simulink subsystem "RoboticArmGeneral7DOF"  (R2022a)
settings: Solver=VariableStepAuto  StartTime=0.0  StopTime=10.0  RelTol=1e-3
undefined symbols (not defined in the file): armAttachOffset, smiData, X, Y, Z
libraries: nesl_utility x227, sm_lib x75
(part 1 of 3)
settings Model: Creator=Andy  LastModifiedBy=Andy

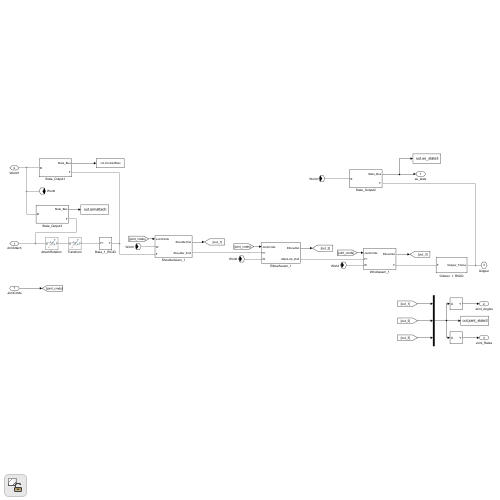
[thumbnail: Simulink's stored preview of the top-level diagram]
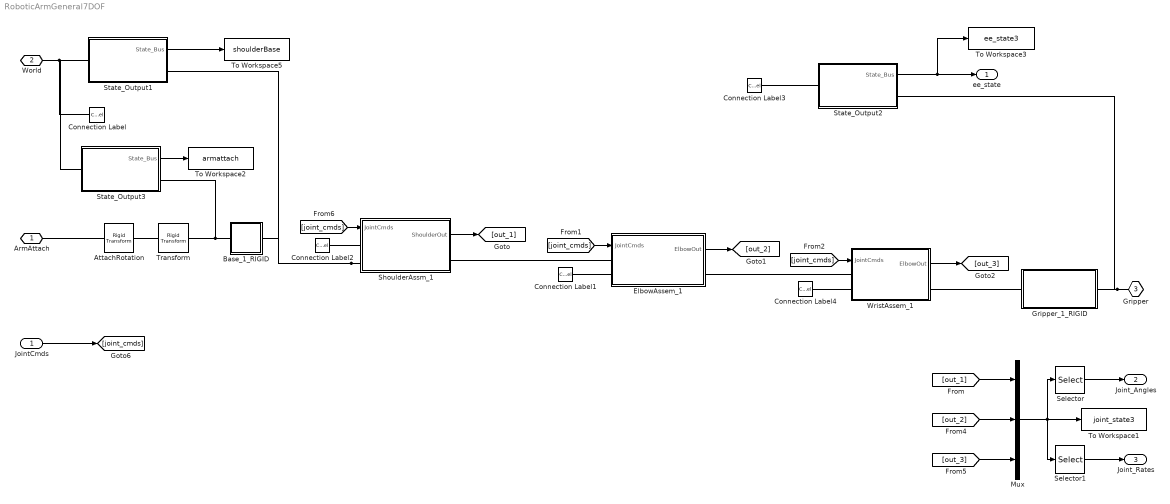
== system RoboticArmGeneral7DOF ==
  JointCmds : Inport
  AttachRotation : sm_lib/Frames and Transforms/Rigid Transform  TranslationMethod=Cartesian  TranslationStandardOffset=0  TranslationLengthUnit=m  TranslationStandardAxis=+Z  TranslationCartesianOffset=armAttachOffset(1).translation  TranslationROffset=0  TranslationROffsetUnits=m  TranslationZOffset=0  TranslationZOffsetUnits=m  TranslationThetaOffset=0  TranslationThetaOffsetUnits=deg  RotationMethod=RotationSequence  RotationAngleUnits=rad  RotationStandardAxis=+Z  RotationAngle=smiData.RigidTransform(21).angle  RotationArbitraryAxis=smiData.RigidTransform(21).axis  FollAlignAxisA=+X  BaseAlignAxisA=+Y  FollAlignAxisB=+Y  BaseAlignAxisB=+Z  RotationSequenceAxes=BaseAxes  RotationSequence=ZYX  RotationSequenceAngles=armAttachOffset(1).orientation  RotationSequenceAnglesUnits=rad  RotationMatrix=[1 0 0; 0 1 0; 0 0 1]
  Base_1_RIGID : Subsystem
  Connection Label{,1..4} (5 alike) : ConnectionLabel  Label=World
  ElbowAssem_1 : Subsystem
  Gripper_1_RIGID : Subsystem
  Mux : Mux  Inputs=3
  Selector : Selector  InputPortWidth=28  IndexOptions=Index vector (dialog)  Indices=[1 5 9 13 17 21 25]  OutputSizes=1
  Selector1 : Selector  InputPortWidth=28  IndexOptions=Index vector (dialog)  Indices=[2 6 10 14 18 22 26]  OutputSizes=1
  ShoulderAssm_1 : Subsystem
  State_Output1 : Subsystem
  State_Output2 : Subsystem
  State_Output3 : Subsystem
  To Workspace1 : ToWorkspace  VariableName=joint_state3  SaveFormat=Timeseries  SampleTime=-1
  To Workspace2 : ToWorkspace  VariableName=armattach  SaveFormat=Timeseries  SampleTime=-1
  To Workspace3 : ToWorkspace  VariableName=ee_state3  SaveFormat=Timeseries  SampleTime=-1
  To Workspace5 : ToWorkspace  VariableName=shoulderBase  SaveFormat=Timeseries  SampleTime=-1
  Transform : sm_lib/Frames and Transforms/Rigid Transform  TranslationMethod=Cartesian  TranslationStandardOffset=0  TranslationLengthUnit=m  TranslationStandardAxis=+Z  TranslationCartesianOffset=smiData.RigidTransform(26).translation  TranslationROffset=0  TranslationROffsetUnits=m  TranslationZOffset=0  TranslationZOffsetUnits=m  TranslationThetaOffset=0  TranslationThetaOffsetUnits=deg  RotationMethod=ArbitraryAxis  RotationAngleUnits=rad  RotationStandardAxis=+Z  RotationAngle=smiData.RigidTransform(26).angle  RotationArbitraryAxis=smiData.RigidTransform(26).axis  FollAlignAxisA=+X  BaseAlignAxisA=+Y  FollAlignAxisB=+Y  BaseAlignAxisB=+Z  RotationSequenceAxes=FollowerAxes  RotationSequence=XYX  RotationSequenceAngles=[0 0 0]  RotationSequenceAnglesUnits=deg  RotationMatrix=[1 0 0; 0 1 0; 0 0 1]
  WristAssem_1 : Subsystem
  ArmAttach : PMIOPort  Side=Left
  World : PMIOPort  Port=2  Side=Left
  Gripper : PMIOPort  Port=3  Side=Right
  ee_state : Outport
  Joint_Angles : Outport  Port=2
  Joint_Rates : Outport  Port=3
  wires:
  Mux/1 -> Selector1/1, Selector/1, To Workspace1/1
  [out_2] -> Mux/2
  [out_3] -> Mux/3
  State_Output1/1(State_Bus) -> To Workspace5/1
  Selector1/1 -> Joint_Rates/1
  ShoulderAssm_1/1(ShoulderOut) -> [out_1]
  [joint_cmds] -> ElbowAssem_1/1(JointCmds)
  Selector/1 -> Joint_Angles/1
  State_Output2/1(State_Bus) -> ee_state/1, To Workspace3/1
  [out_1] -> Mux/1
  [joint_cmds] -> WristAssem_1/1(JointCmds)
  JointCmds/1 -> [joint_cmds]
  ElbowAssem_1/1(ElbowOut) -> [out_2]
  State_Output3/1(State_Bus) -> To Workspace2/1
  [joint_cmds] -> ShoulderAssm_1/1(JointCmds)
  WristAssem_1/1(ElbowOut) -> [out_3]
  connections:
  ShoulderAssm_1/LConn2 -- State_Output1/RConn1 -- Base_1_RIGID/RConn1
  World/RConn1 -- Connection Label/LConn1 -- State_Output3/LConn1 -- State_Output1/LConn1
  Gripper/RConn1 -- State_Output2/RConn1 -- Gripper_1_RIGID/RConn1
  State_Output3/RConn1 -- Base_1_RIGID/LConn1 -- Transform/RConn1
  ArmAttach/RConn1 -- AttachRotation/LConn1
  AttachRotation/RConn1 -- Transform/LConn1
  Connection Label2/LConn1 -- ShoulderAssm_1/LConn1
  Connection Label3/LConn1 -- State_Output2/LConn1
  Connection Label4/LConn1 -- WristAssem_1/LConn2
  ElbowAssem_1/LConn1 -- ShoulderAssm_1/RConn1
  Connection Label1/LConn1 -- ElbowAssem_1/LConn2
  ElbowAssem_1/RConn1 -- WristAssem_1/LConn1
  WristAssem_1/RConn1 -- Gripper_1_RIGID/LConn1

== system RoboticArmGeneral7DOF/Base_1_RIGID ==
  ReferenceFrame : sm_lib/Frames and Transforms/Reference Frame
  Solid : sm_lib/Body Elements/File Solid  ExtGeomFileName=Base_Default_sldprt.STEP  UnitType=FromFile  ExtGeomFileUnits=m  StepReaderType=HEX  ExportConvexHullGeometry=off  InertiaType=Custom  Mass=smiData.Solid(11).mass  MassUnits=kg  CenterOfMass=smiData.Solid(11).CoM  CenterOfMassUnits=m  MomentsOfInertia=smiData.Solid(11).MoI  MomentsOfInertiaUnits=kg*m^2  ProductsOfInertia=smiData.Solid(11).PoI  ProductsOfInertiaUnits=kg*m^2  BasedOnType=DensityFromFile  Density=1000  DensityUnits=kg/m^3  DoExposeReferenceFrame=on  SerializedFrames=<Frames/>  GraphicType=FromGeometry  MarkerShape=Sphere  MarkerSize=10  GraphicVisPropType=SimpleVisualProperties  GraphicDiffuseColor=smiData.Solid(11).color  GraphicSpecularColor=[0.5 0.5 0.5 1.0]  GraphicAmbientColor=[0.15 0.15 0.15 1.0]  GraphicEmissiveColor=[0.0 0.0 0.0 1.0]  GraphicShininess=75  GraphicOpacity=smiData.Solid(11).opacity
  Transform : sm_lib/Frames and Transforms/Rigid Transform  TranslationMethod=Cartesian  TranslationStandardOffset=0  TranslationLengthUnit=m  TranslationStandardAxis=+Z  TranslationCartesianOffset=smiData.RigidTransform(16).translation  TranslationROffset=0  TranslationROffsetUnits=m  TranslationZOffset=0  TranslationZOffsetUnits=m  TranslationThetaOffset=0  TranslationThetaOffsetUnits=deg  RotationMethod=ArbitraryAxis  RotationAngleUnits=rad  RotationStandardAxis=+Z  RotationAngle=smiData.RigidTransform(16).angle  RotationArbitraryAxis=smiData.RigidTransform(16).axis  FollAlignAxisA=+X  BaseAlignAxisA=+Y  FollAlignAxisB=+Y  BaseAlignAxisB=+Z  RotationSequenceAxes=FollowerAxes  RotationSequence=XYX  RotationSequenceAngles=[0 0 0]  RotationSequenceAnglesUnits=deg  RotationMatrix=[1 0 0; 0 1 0; 0 0 1]
  F : PMIOPort  Side=Right
  F1 : PMIOPort  Port=2  Side=Left
  connections:
  Transform/RConn1 -- F/RConn1
  F1/RConn1 -- Transform/LConn1 -- ReferenceFrame/RConn1 -- Solid/RConn1

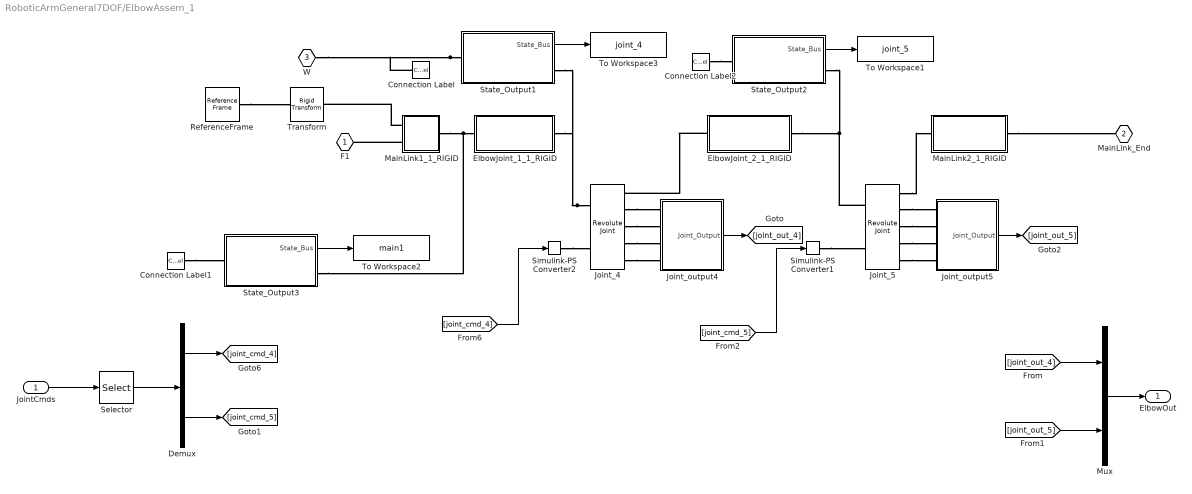
== system RoboticArmGeneral7DOF/ElbowAssem_1 ==
  JointCmds : Inport
  Connection Label : ConnectionLabel  Label=World
  Connection Label1 : ConnectionLabel  Label=World
  Connection Label2 : ConnectionLabel  Label=World
  Demux : Demux  Outputs=2
  ElbowJoint_1_1_RIGID : Subsystem
  ElbowJoint_2_1_RIGID : Subsystem
  Joint_4 : sm_lib/Joints/Revolute Joint  JointMode=Normal  SenseConstraintForce=off  SenseConstraintForceX=off  SenseConstraintForceY=off  SenseConstraintForceZ=off  SenseConstraintTorque=off  SenseConstraintTorqueX=off  SenseConstraintTorqueY=off  SenseConstraintTorqueZ=off  SenseTotalForce=off  SenseTotalForceX=off  SenseTotalForceY=off  SenseTotalForceZ=off  SenseTotalTorque=on  SenseTotalTorqueX=off  SenseTotalTorqueY=off  SenseTotalTorqueZ=off  CompositeWrenchDir=FollowerOnBase  CompositeWrenchFrame=BaseFrame  EquilibriumPosition=0  EquilibriumPositionUnits=deg  SpringStiffness=0  SpringStiffnessUnits=N*m/deg  DampingCoefficient=0  DampingCoefficientUnits=N*m/(deg/s)  TorqueActuationMode=InputTorque  MotionActuationMode=ComputedMotion  SensePosition=on  SenseVelocity=on  SenseAcceleration=on  SenseTorqueForce=off  SenseLowerLimitTorqueForce=off  SenseUpperLimitTorqueForce=off  LowerLimitSpecify=off  LowerLimitBound=-90  LowerLimitBoundUnits=deg  LowerLimitStiffness=1e4  LowerLimitStiffnessUnits=N*m/deg  LowerLimitDamping=10  LowerLimitDampingUnits=N*m/(deg/s)  LowerLimitTransitionRegionWidth=0.1  LowerLimitTransitionRegionWidthUnits=deg  UpperLimitSpecify=off  UpperLimitBound=90  UpperLimitBoundUnits=deg  UpperLimitStiffness=1e4  UpperLimitStiffnessUnits=N*m/deg  UpperLimitDamping=10  UpperLimitDampingUnits=N*m/(deg/s)  UpperLimitTransitionRegionWidth=0.1  UpperLimitTransitionRegionWidthUnits=deg  PositionTargetSpecify=on  PositionTargetPriority=Low  PositionTargetValue=smiData.RevoluteJoint(4).Rz.Pos  PositionTargetValueUnits=deg  VelocityTargetSpecify=off  VelocityTargetPriority=High  VelocityTargetValue=0  VelocityTargetValueUnits=deg/s
  Joint_5 : sm_lib/Joints/Revolute Joint  JointMode=Normal  SenseConstraintForce=off  SenseConstraintForceX=off  SenseConstraintForceY=off  SenseConstraintForceZ=off  SenseConstraintTorque=off  SenseConstraintTorqueX=off  SenseConstraintTorqueY=off  SenseConstraintTorqueZ=off  SenseTotalForce=off  SenseTotalForceX=off  SenseTotalForceY=off  SenseTotalForceZ=off  SenseTotalTorque=on  SenseTotalTorqueX=off  SenseTotalTorqueY=off  SenseTotalTorqueZ=off  CompositeWrenchDir=FollowerOnBase  CompositeWrenchFrame=BaseFrame  EquilibriumPosition=0  EquilibriumPositionUnits=deg  SpringStiffness=0  SpringStiffnessUnits=N*m/deg  DampingCoefficient=0  DampingCoefficientUnits=N*m/(deg/s)  TorqueActuationMode=InputTorque  MotionActuationMode=ComputedMotion  SensePosition=on  SenseVelocity=on  SenseAcceleration=on  SenseTorqueForce=off  SenseLowerLimitTorqueForce=off  SenseUpperLimitTorqueForce=off  LowerLimitSpecify=off  LowerLimitBound=-90  LowerLimitBoundUnits=deg  LowerLimitStiffness=1e4  LowerLimitStiffnessUnits=N*m/deg  LowerLimitDamping=10  LowerLimitDampingUnits=N*m/(deg/s)  LowerLimitTransitionRegionWidth=0.1  LowerLimitTransitionRegionWidthUnits=deg  UpperLimitSpecify=off  UpperLimitBound=90  UpperLimitBoundUnits=deg  UpperLimitStiffness=1e4  UpperLimitStiffnessUnits=N*m/deg  UpperLimitDamping=10  UpperLimitDampingUnits=N*m/(deg/s)  UpperLimitTransitionRegionWidth=0.1  UpperLimitTransitionRegionWidthUnits=deg  PositionTargetSpecify=on  PositionTargetPriority=Low  PositionTargetValue=smiData.RevoluteJoint(5).Rz.Pos  PositionTargetValueUnits=deg  VelocityTargetSpecify=off  VelocityTargetPriority=High  VelocityTargetValue=0  VelocityTargetValueUnits=deg/s
  Joint_output4 : Subsystem
  Joint_output5 : Subsystem
  MainLink1_1_RIGID : Subsystem
  MainLink2_1_RIGID : Subsystem
  Mux : Mux  Inputs=2
  ReferenceFrame : sm_lib/Frames and Transforms/Reference Frame
  Selector : Selector  InputPortWidth=7  IndexOptions=Index vector (dialog)  Indices=[4 5]  OutputSizes=1
  Simulink-PS Converter1 : nesl_utility/Simulink-PS Converter  PhysicalDomain=network_engine_domain  SubClassName=ps_input  LeftPortType=input  RightPortType=output  PseudoPeriodic=off  Frequencies=[]  NoiseDistribution=none  NoiseParameters=[]  Unit=1  AffineConversion=off  FilteringAndDerivatives=filter  SimscapeFilterOrder=2  InputFilterTimeConstant=0.001  UdotUserProvided=0
      settings: SourceProductBaseCode=SS,PW,VE
  Simulink-PS Converter2 : nesl_utility/Simulink-PS Converter  PhysicalDomain=network_engine_domain  SubClassName=ps_input  LeftPortType=input  RightPortType=output  PseudoPeriodic=off  Frequencies=[]  NoiseDistribution=none  NoiseParameters=[]  Unit=1  AffineConversion=off  FilteringAndDerivatives=filter  SimscapeFilterOrder=2  InputFilterTimeConstant=0.001  UdotUserProvided=0
      settings: SourceProductBaseCode=SS,PW,VE
  State_Output1 : Subsystem
  State_Output2 : Subsystem
  State_Output3 : Subsystem
  To Workspace1 : ToWorkspace  VariableName=joint_5  SaveFormat=Timeseries  SampleTime=-1
  To Workspace2 : ToWorkspace  VariableName=main1  SaveFormat=Timeseries  SampleTime=-1
  To Workspace3 : ToWorkspace  VariableName=joint_4  SaveFormat=Timeseries  SampleTime=-1
  Transform : sm_lib/Frames and Transforms/Rigid Transform  TranslationMethod=Cartesian  TranslationStandardOffset=0  TranslationLengthUnit=m  TranslationStandardAxis=+Z  TranslationCartesianOffset=smiData.RigidTransform(23).translation  TranslationROffset=0  TranslationROffsetUnits=m  TranslationZOffset=0  TranslationZOffsetUnits=m  TranslationThetaOffset=0  TranslationThetaOffsetUnits=deg  RotationMethod=ArbitraryAxis  RotationAngleUnits=rad  RotationStandardAxis=+Z  RotationAngle=smiData.RigidTransform(23).angle  RotationArbitraryAxis=smiData.RigidTransform(23).axis  FollAlignAxisA=+X  BaseAlignAxisA=+Y  FollAlignAxisB=+Y  BaseAlignAxisB=+Z  RotationSequenceAxes=FollowerAxes  RotationSequence=XYX  RotationSequenceAngles=[0 0 0]  RotationSequenceAnglesUnits=deg  RotationMatrix=[1 0 0; 0 1 0; 0 0 1]
  F1 : PMIOPort  Side=Left
  MainLink_End : PMIOPort  Port=2  Side=Right
  W : PMIOPort  Port=3  Side=Left
  ElbowOut : Outport
  wires:
  State_Output3/1(State_Bus) -> To Workspace2/1
  Joint_output5/1(Joint_Output) -> [joint_out_5]
  [joint_cmd_5] -> Simulink-PS Converter1/1
  State_Output2/1(State_Bus) -> To Workspace1/1
  State_Output1/1(State_Bus) -> To Workspace3/1
  [joint_cmd_4] -> Simulink-PS Converter2/1
  Joint_output4/1(Joint_Output) -> [joint_out_4]
  [joint_out_5] -> Mux/2
  Demux/2 -> [joint_cmd_5]
  Mux/1 -> ElbowOut/1
  Selector/1 -> Demux/1
  JointCmds/1 -> Selector/1
  Demux/1 -> [joint_cmd_4]
  [joint_out_4] -> Mux/1
  connections:
  Connection Label1/LConn1 -- State_Output3/LConn1
  State_Output1/LConn1 -- Connection Label/LConn1 -- W/RConn1
  Joint_5/RConn3 -- Joint_output5/LConn2
  Joint_5/RConn2 -- Joint_output5/LConn1
  Joint_5/RConn1 -- MainLink2_1_RIGID/LConn1
  Joint_5/RConn4 -- Joint_output5/LConn3
  Joint_5/RConn5 -- Joint_output5/LConn4
  Simulink-PS Converter1/RConn1 -- Joint_5/LConn2
  ElbowJoint_2_1_RIGID/LConn1 -- Joint_4/RConn1
  Joint_4/LConn1 -- State_Output1/RConn1 -- ElbowJoint_1_1_RIGID/RConn1
  State_Output3/RConn1 -- MainLink1_1_RIGID/RConn1 -- ElbowJoint_1_1_RIGID/LConn1
  Connection Label2/LConn1 -- State_Output2/LConn1
  Joint_4/RConn2 -- Joint_output4/LConn1
  Joint_4/RConn4 -- Joint_output4/LConn3
  Joint_4/RConn3 -- Joint_output4/LConn2
  Joint_4/RConn5 -- Joint_output4/LConn4
  Simulink-PS Converter2/RConn1 -- Joint_4/LConn2
  ReferenceFrame/RConn1 -- Transform/LConn1
  MainLink1_1_RIGID/LConn1 -- Transform/RConn1
  MainLink1_1_RIGID/LConn2 -- F1/RConn1
  MainLink2_1_RIGID/RConn1 -- MainLink_End/RConn1
  State_Output2/RConn1 -- Joint_5/LConn1 -- ElbowJoint_2_1_RIGID/RConn1

== system RoboticArmGeneral7DOF/Gripper_1_RIGID ==
  ReferenceFrame : sm_lib/Frames and Transforms/Reference Frame
  Solid : sm_lib/Body Elements/File Solid  ExtGeomFileName=Gripper2_Default_sldprt.STEP  UnitType=FromFile  ExtGeomFileUnits=m  StepReaderType=HEX  ExportConvexHullGeometry=off  InertiaType=Custom  Mass=smiData.Solid(12).mass  MassUnits=kg  CenterOfMass=smiData.Solid(12).CoM  CenterOfMassUnits=m  MomentsOfInertia=smiData.Solid(12).MoI  MomentsOfInertiaUnits=kg*m^2  ProductsOfInertia=smiData.Solid(12).PoI  ProductsOfInertiaUnits=kg*m^2  BasedOnType=DensityFromFile  Density=1000  DensityUnits=kg/m^3  DoExposeReferenceFrame=on  SerializedFrames=<Frames/>  GraphicType=FromGeometry  MarkerShape=Sphere  MarkerSize=10  GraphicVisPropType=SimpleVisualProperties  GraphicDiffuseColor=smiData.Solid(12).color  GraphicSpecularColor=[0.5 0.5 0.5 1.0]  GraphicAmbientColor=[0.15 0.15 0.15 1.0]  GraphicEmissiveColor=[0.0 0.0 0.0 1.0]  GraphicShininess=75  GraphicOpacity=smiData.Solid(12).opacity
  Transform : sm_lib/Frames and Transforms/Rigid Transform  TranslationMethod=Cartesian  TranslationStandardOffset=0  TranslationLengthUnit=m  TranslationStandardAxis=+Z  TranslationCartesianOffset=smiData.RigidTransform(18).translation  TranslationROffset=0  TranslationROffsetUnits=m  TranslationZOffset=0  TranslationZOffsetUnits=m  TranslationThetaOffset=0  TranslationThetaOffsetUnits=deg  RotationMethod=ArbitraryAxis  RotationAngleUnits=rad  RotationStandardAxis=+Z  RotationAngle=smiData.RigidTransform(18).angle  RotationArbitraryAxis=smiData.RigidTransform(18).axis  FollAlignAxisA=+X  BaseAlignAxisA=+Y  FollAlignAxisB=+Y  BaseAlignAxisB=+Z  RotationSequenceAxes=FollowerAxes  RotationSequence=XYX  RotationSequenceAngles=[0 0 0]  RotationSequenceAnglesUnits=deg  RotationMatrix=[1 0 0; 0 1 0; 0 0 1]
  Transform1 : sm_lib/Frames and Transforms/Rigid Transform  TranslationMethod=Cartesian  TranslationStandardOffset=0  TranslationLengthUnit=m  TranslationStandardAxis=+Z  TranslationCartesianOffset=smiData.RigidTransform(27).translation  TranslationROffset=0  TranslationROffsetUnits=m  TranslationZOffset=0  TranslationZOffsetUnits=m  TranslationThetaOffset=0  TranslationThetaOffsetUnits=deg  RotationMethod=ArbitraryAxis  RotationAngleUnits=rad  RotationStandardAxis=+Z  RotationAngle=smiData.RigidTransform(27).angle  RotationArbitraryAxis=smiData.RigidTransform(27).axis  FollAlignAxisA=+X  BaseAlignAxisA=+Y  FollAlignAxisB=+Y  BaseAlignAxisB=+Z  RotationSequenceAxes=FollowerAxes  RotationSequence=XYX  RotationSequenceAngles=[0 0 0]  RotationSequenceAnglesUnits=deg  RotationMatrix=[1 0 0; 0 1 0; 0 0 1]
  F : PMIOPort  Side=Left
  Gripper_Frame : PMIOPort  Port=2  Side=Right
  connections:
  Gripper_Frame/RConn1 -- Transform1/RConn1
  Transform/RConn1 -- F/RConn1
  Transform/LConn1 -- Transform1/LConn1 -- ReferenceFrame/RConn1 -- Solid/RConn1

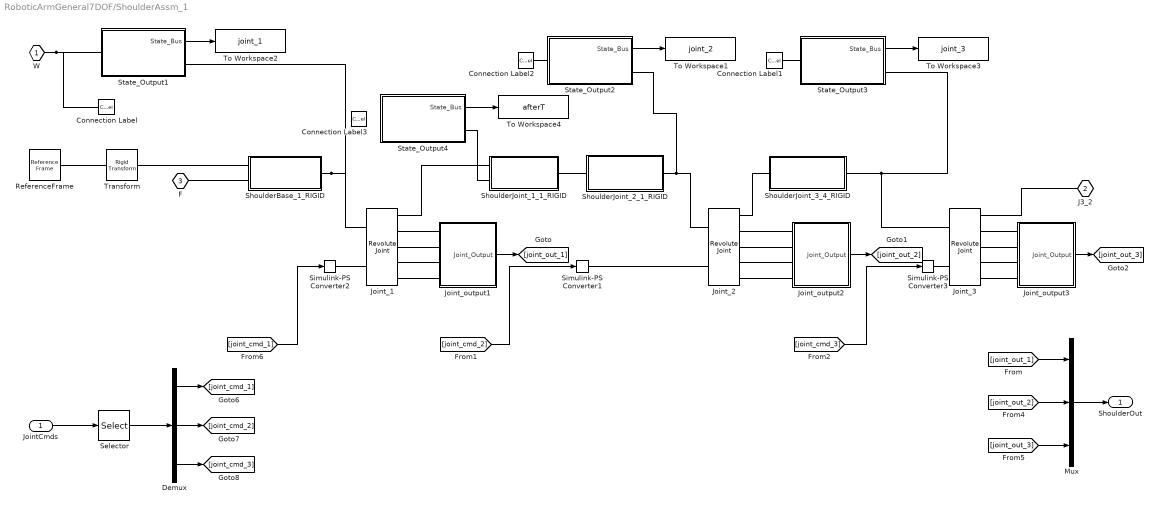
== system RoboticArmGeneral7DOF/ShoulderAssm_1 ==
  JointCmds : Inport
  Connection Label{,1..3} (4 alike) : ConnectionLabel  Label=World
  Demux : Demux  Outputs=3
  Joint_1 : sm_lib/Joints/Revolute Joint  JointMode=Normal  SenseConstraintForce=off  SenseConstraintForceX=off  SenseConstraintForceY=off  SenseConstraintForceZ=off  SenseConstraintTorque=off  SenseConstraintTorqueX=off  SenseConstraintTorqueY=off  SenseConstraintTorqueZ=off  SenseTotalForce=off  SenseTotalForceX=off  SenseTotalForceY=off  SenseTotalForceZ=off  SenseTotalTorque=on  SenseTotalTorqueX=off  SenseTotalTorqueY=off  SenseTotalTorqueZ=off  CompositeWrenchDir=FollowerOnBase  CompositeWrenchFrame=BaseFrame  EquilibriumPosition=0  EquilibriumPositionUnits=deg  SpringStiffness=0  SpringStiffnessUnits=N*m/deg  DampingCoefficient=0  DampingCoefficientUnits=N*m/(deg/s)  TorqueActuationMode=InputTorque  MotionActuationMode=ComputedMotion  SensePosition=on  SenseVelocity=on  SenseAcceleration=on  SenseTorqueForce=off  SenseLowerLimitTorqueForce=off  SenseUpperLimitTorqueForce=off  LowerLimitSpecify=off  LowerLimitBound=-90  LowerLimitBoundUnits=deg  LowerLimitStiffness=1e4  LowerLimitStiffnessUnits=N*m/deg  LowerLimitDamping=10  LowerLimitDampingUnits=N*m/(deg/s)  LowerLimitTransitionRegionWidth=0.1  LowerLimitTransitionRegionWidthUnits=deg  UpperLimitSpecify=off  UpperLimitBound=90  UpperLimitBoundUnits=deg  UpperLimitStiffness=1e4  UpperLimitStiffnessUnits=N*m/deg  UpperLimitDamping=10  UpperLimitDampingUnits=N*m/(deg/s)  UpperLimitTransitionRegionWidth=0.1  UpperLimitTransitionRegionWidthUnits=deg  PositionTargetSpecify=on  PositionTargetPriority=Low  PositionTargetValue=smiData.RevoluteJoint(1).Rz.Pos  PositionTargetValueUnits=deg  VelocityTargetSpecify=off  VelocityTargetPriority=High  VelocityTargetValue=0  VelocityTargetValueUnits=deg/s
  Joint_2 : sm_lib/Joints/Revolute Joint  JointMode=Normal  SenseConstraintForce=off  SenseConstraintForceX=off  SenseConstraintForceY=off  SenseConstraintForceZ=off  SenseConstraintTorque=off  SenseConstraintTorqueX=off  SenseConstraintTorqueY=off  SenseConstraintTorqueZ=off  SenseTotalForce=off  SenseTotalForceX=off  SenseTotalForceY=off  SenseTotalForceZ=off  SenseTotalTorque=on  SenseTotalTorqueX=off  SenseTotalTorqueY=off  SenseTotalTorqueZ=off  CompositeWrenchDir=FollowerOnBase  CompositeWrenchFrame=BaseFrame  EquilibriumPosition=0  EquilibriumPositionUnits=deg  SpringStiffness=0  SpringStiffnessUnits=N*m/deg  DampingCoefficient=0  DampingCoefficientUnits=N*m/(deg/s)  TorqueActuationMode=InputTorque  MotionActuationMode=ComputedMotion  SensePosition=on  SenseVelocity=on  SenseAcceleration=on  SenseTorqueForce=off  SenseLowerLimitTorqueForce=off  SenseUpperLimitTorqueForce=off  LowerLimitSpecify=off  LowerLimitBound=-90  LowerLimitBoundUnits=deg  LowerLimitStiffness=1e4  LowerLimitStiffnessUnits=N*m/deg  LowerLimitDamping=10  LowerLimitDampingUnits=N*m/(deg/s)  LowerLimitTransitionRegionWidth=0.1  LowerLimitTransitionRegionWidthUnits=deg  UpperLimitSpecify=off  UpperLimitBound=90  UpperLimitBoundUnits=deg  UpperLimitStiffness=1e4  UpperLimitStiffnessUnits=N*m/deg  UpperLimitDamping=10  UpperLimitDampingUnits=N*m/(deg/s)  UpperLimitTransitionRegionWidth=0.1  UpperLimitTransitionRegionWidthUnits=deg  PositionTargetSpecify=on  PositionTargetPriority=Low  PositionTargetValue=smiData.RevoluteJoint(2).Rz.Pos  PositionTargetValueUnits=deg  VelocityTargetSpecify=off  VelocityTargetPriority=High  VelocityTargetValue=0  VelocityTargetValueUnits=deg/s
  Joint_3 : sm_lib/Joints/Revolute Joint  JointMode=Normal  SenseConstraintForce=off  SenseConstraintForceX=off  SenseConstraintForceY=off  SenseConstraintForceZ=off  SenseConstraintTorque=off  SenseConstraintTorqueX=off  SenseConstraintTorqueY=off  SenseConstraintTorqueZ=off  SenseTotalForce=off  SenseTotalForceX=off  SenseTotalForceY=off  SenseTotalForceZ=off  SenseTotalTorque=on  SenseTotalTorqueX=off  SenseTotalTorqueY=off  SenseTotalTorqueZ=off  CompositeWrenchDir=FollowerOnBase  CompositeWrenchFrame=BaseFrame  EquilibriumPosition=0  EquilibriumPositionUnits=deg  SpringStiffness=0  SpringStiffnessUnits=N*m/deg  DampingCoefficient=0  DampingCoefficientUnits=N*m/(deg/s)  TorqueActuationMode=InputTorque  MotionActuationMode=ComputedMotion  SensePosition=on  SenseVelocity=on  SenseAcceleration=on  SenseTorqueForce=off  SenseLowerLimitTorqueForce=off  SenseUpperLimitTorqueForce=off  LowerLimitSpecify=off  LowerLimitBound=-90  LowerLimitBoundUnits=deg  LowerLimitStiffness=1e4  LowerLimitStiffnessUnits=N*m/deg  LowerLimitDamping=10  LowerLimitDampingUnits=N*m/(deg/s)  LowerLimitTransitionRegionWidth=0.1  LowerLimitTransitionRegionWidthUnits=deg  UpperLimitSpecify=off  UpperLimitBound=90  UpperLimitBoundUnits=deg  UpperLimitStiffness=1e4  UpperLimitStiffnessUnits=N*m/deg  UpperLimitDamping=10  UpperLimitDampingUnits=N*m/(deg/s)  UpperLimitTransitionRegionWidth=0.1  UpperLimitTransitionRegionWidthUnits=deg  PositionTargetSpecify=on  PositionTargetPriority=Low  PositionTargetValue=smiData.RevoluteJoint(3).Rz.Pos  PositionTargetValueUnits=deg  VelocityTargetSpecify=off  VelocityTargetPriority=High  VelocityTargetValue=0  VelocityTargetValueUnits=deg/s
  Joint_output1 : Subsystem
  Joint_output2 : Subsystem
  Joint_output3 : Subsystem
  Mux : Mux  Inputs=3
  ReferenceFrame : sm_lib/Frames and Transforms/Reference Frame
  Selector : Selector  InputPortWidth=7  IndexOptions=Index vector (dialog)  Indices=[1 2 3]  OutputSizes=1
  ShoulderBase_1_RIGID : Subsystem
  ShoulderJoint_1_1_RIGID : Subsystem
  ShoulderJoint_2_1_RIGID : Subsystem
  ShoulderJoint_3_4_RIGID : Subsystem
  Simulink-PS Converter1 : nesl_utility/Simulink-PS Converter  PhysicalDomain=network_engine_domain  SubClassName=ps_input  LeftPortType=input  RightPortType=output  PseudoPeriodic=off  Frequencies=[]  NoiseDistribution=none  NoiseParameters=[]  Unit=1  AffineConversion=off  FilteringAndDerivatives=filter  SimscapeFilterOrder=2  InputFilterTimeConstant=0.001  UdotUserProvided=0
      settings: SourceProductBaseCode=SS,PW,VE
  Simulink-PS Converter2 : nesl_utility/Simulink-PS Converter  PhysicalDomain=network_engine_domain  SubClassName=ps_input  LeftPortType=input  RightPortType=output  PseudoPeriodic=off  Frequencies=[]  NoiseDistribution=none  NoiseParameters=[]  Unit=1  AffineConversion=off  FilteringAndDerivatives=filter  SimscapeFilterOrder=2  InputFilterTimeConstant=0.001  UdotUserProvided=0
      settings: SourceProductBaseCode=SS,PW,VE
  Simulink-PS Converter3 : nesl_utility/Simulink-PS Converter  PhysicalDomain=network_engine_domain  SubClassName=ps_input  LeftPortType=input  RightPortType=output  PseudoPeriodic=off  Frequencies=[]  NoiseDistribution=none  NoiseParameters=[]  Unit=1  AffineConversion=off  FilteringAndDerivatives=filter  SimscapeFilterOrder=2  InputFilterTimeConstant=0.001  UdotUserProvided=0
      settings: SourceProductBaseCode=SS,PW,VE
  State_Output1 : Subsystem
  State_Output2 : Subsystem
  State_Output3 : Subsystem
  State_Output4 : Subsystem
  To Workspace1 : ToWorkspace  VariableName=joint_2  SaveFormat=Timeseries  SampleTime=-1
  To Workspace2 : ToWorkspace  VariableName=joint_1  SaveFormat=Timeseries  SampleTime=-1
  To Workspace3 : ToWorkspace  VariableName=joint_3  SaveFormat=Timeseries  SampleTime=-1
  To Workspace4 : ToWorkspace  VariableName=afterT  SaveFormat=Timeseries  SampleTime=-1
  Transform : sm_lib/Frames and Transforms/Rigid Transform  TranslationMethod=Cartesian  TranslationStandardOffset=0  TranslationLengthUnit=m  TranslationStandardAxis=+Z  TranslationCartesianOffset=smiData.RigidTransform(25).translation  TranslationROffset=0  TranslationROffsetUnits=m  TranslationZOffset=0  TranslationZOffsetUnits=m  TranslationThetaOffset=0  TranslationThetaOffsetUnits=deg  RotationMethod=ArbitraryAxis  RotationAngleUnits=rad  RotationStandardAxis=+Z  RotationAngle=smiData.RigidTransform(25).angle  RotationArbitraryAxis=smiData.RigidTransform(25).axis  FollAlignAxisA=+X  BaseAlignAxisA=+Y  FollAlignAxisB=+Y  BaseAlignAxisB=+Z  RotationSequenceAxes=FollowerAxes  RotationSequence=XYX  RotationSequenceAngles=[0 0 0]  RotationSequenceAnglesUnits=deg  RotationMatrix=[1 0 0; 0 1 0; 0 0 1]
  W : PMIOPort  Side=Left
  J3_2 : PMIOPort  Port=2  Side=Right
  F : PMIOPort  Port=3  Side=Left
  ShoulderOut : Outport
  wires:
  State_Output4/1(State_Bus) -> To Workspace4/1
  State_Output3/1(State_Bus) -> To Workspace3/1
  Mux/1 -> ShoulderOut/1
  [joint_out_1] -> Mux/1
  [joint_out_3] -> Mux/3
  [joint_out_2] -> Mux/2
  Joint_output3/1(Joint_Output) -> [joint_out_3]
  Joint_output2/1(Joint_Output) -> [joint_out_2]
  [joint_cmd_3] -> Simulink-PS Converter3/1
  State_Output2/1(State_Bus) -> To Workspace1/1
  State_Output1/1(State_Bus) -> To Workspace2/1
  [joint_cmd_2] -> Simulink-PS Converter1/1
  Joint_output1/1(Joint_Output) -> [joint_out_1]
  [joint_cmd_1] -> Simulink-PS Converter2/1
  JointCmds/1 -> Selector/1
  Demux/2 -> [joint_cmd_2]
  Demux/1 -> [joint_cmd_1]
  Selector/1 -> Demux/1
  Demux/3 -> [joint_cmd_3]
  connections:
  Joint_3/RConn1 -- J3_2/RConn1
  ShoulderJoint_3_4_RIGID/LConn1 -- Joint_2/RConn1
  State_Output2/RConn1 -- Joint_2/LConn1 -- ShoulderJoint_2_1_RIGID/RConn1
  State_Output4/RConn1 -- ShoulderJoint_1_1_RIGID/LConn2
  Connection Label1/LConn1 -- State_Output3/LConn1
  Simulink-PS Converter3/RConn1 -- Joint_3/LConn2
  Joint_output2/LConn3 -- Joint_2/RConn4
  Joint_3/RConn4 -- Joint_output3/LConn3
  Joint_3/RConn2 -- Joint_output3/LConn1
  Joint_3/RConn3 -- Joint_output3/LConn2
  Joint_output2/LConn4 -- Joint_2/RConn5
  Joint_output2/LConn2 -- Joint_2/RConn3
  Joint_output2/LConn1 -- Joint_2/RConn2
  Joint_3/RConn5 -- Joint_output3/LConn4
  Connection Label2/LConn1 -- State_Output2/LConn1
  ShoulderJoint_2_1_RIGID/LConn1 -- ShoulderJoint_1_1_RIGID/RConn1
  Simulink-PS Converter1/RConn1 -- Joint_2/LConn2
  Joint_output1/LConn4 -- Joint_1/RConn5
  Joint_1/RConn3 -- Joint_output1/LConn2
  Joint_output1/LConn1 -- Joint_1/RConn2
  Joint_output1/LConn3 -- Joint_1/RConn4
  Joint_1/LConn2 -- Simulink-PS Converter2/RConn1
  W/RConn1 -- Connection Label/LConn1 -- State_Output1/LConn1
  ReferenceFrame/RConn1 -- Transform/LConn1
  ShoulderBase_1_RIGID/LConn1 -- Transform/RConn1
  State_Output3/RConn1 -- ShoulderJoint_3_4_RIGID/RConn1 -- Joint_3/LConn1
  ShoulderBase_1_RIGID/LConn2 -- F/RConn1
  Joint_1/RConn1 -- ShoulderJoint_1_1_RIGID/LConn1
  ShoulderBase_1_RIGID/RConn1 -- State_Output1/RConn1 -- Joint_1/LConn1

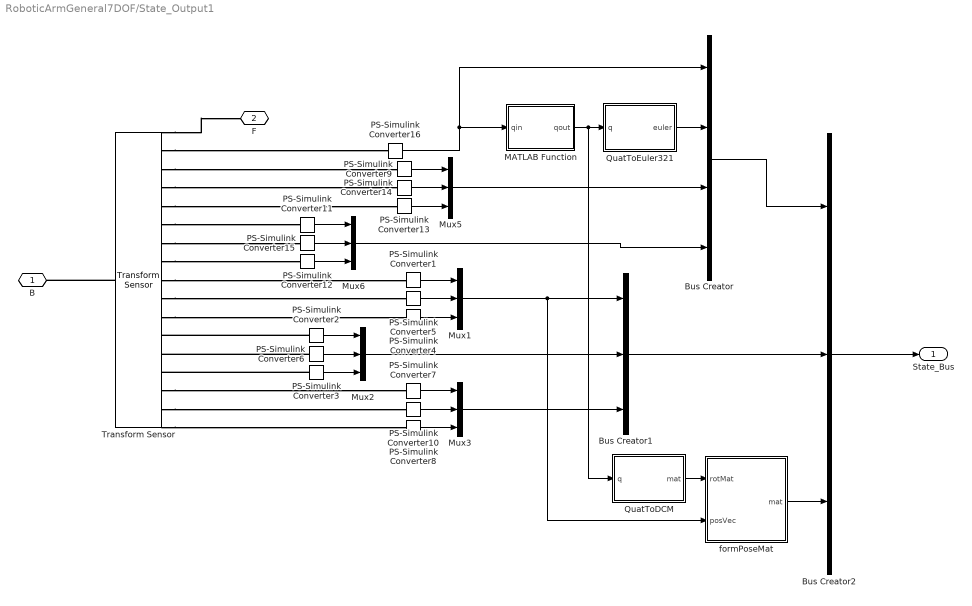
== system RoboticArmGeneral7DOF/State_Output1 ==
  Bus Creator : BusCreator  Inputs=4  OutDataTypeStr=Bus: RotStateBus
      settings: InheritFromInputs=off
  Bus Creator1 : BusCreator  Inputs=3  OutDataTypeStr=Bus: TransStateBus
      settings: InheritFromInputs=off
  Bus Creator2 : BusCreator  Inputs=3  OutDataTypeStr=Bus: StateBus
      settings: InheritFromInputs=off
  MATLAB Function : MATLAB Function  TreatAsAtomicUnit=on
  Mux{1..3,5..6} (5 alike) : Mux  Inputs=3
  PS-Simulink Converter{1..16} (16 alike) : nesl_utility/PS-Simulink Converter  PhysicalDomain=network_engine_domain  SubClassName=ps_output  LeftPortType=input  RightPortType=output  PseudoPeriodic=off  Frequencies=[]  VectorFormat=1-D array  Unit=inherit  AffineConversion=off
      settings: SourceProductBaseCode=SS,PW,VE
  QuatToDCM : MATLAB Function  TreatAsAtomicUnit=on
  QuatToEuler321 : MATLAB Function  TreatAsAtomicUnit=on
  Transform Sensor : sm_lib/Frames and Transforms/Transform Sensor  MeasurementFrame=World  SenseAngle=off  SenseAxis=off  SenseAngle1=off  SenseAngle2=off  SenseAngle3=off  SenseQ=on  SenseR=off  SenseOmegaX=on  SenseOmegaY=on  SenseOmegaZ=on  SenseOmega1=off  SenseOmega2=off  SenseOmega3=off  SenseQDot=off  SenseRDot=off  SenseAlphaX=on  SenseAlphaY=on  SenseAlphaZ=on  SenseAlpha1=off  SenseAlpha2=off  SenseAlpha3=off  SenseQDDot=off  SenseRDDot=off  SenseX=on  SenseY=on  SenseZ=on  SenseRad=off  SenseAzim=off  SenseDist=off  SenseInc=off  SenseXDot=on  SenseYDot=on  SenseZDot=on  SenseRadDot=off  SenseAzimDot=off  SenseDistDot=off  SenseIncDot=off  SenseXDDot=on  SenseYDDot=on  SenseZDDot=on  SenseRadDDot=off  SenseAzimDDot=off  SenseDistDDot=off  SenseIncDDot=off
  formPoseMat : MATLAB Function  TreatAsAtomicUnit=on
  B : PMIOPort  Side=Left
  F : PMIOPort  Port=2  Side=Right
  State_Bus : Outport
  wires:
  PS-Simulink Converter4/1 -> Mux1/3
  PS-Simulink Converter5/1 -> Mux1/2
  PS-Simulink Converter1/1 -> Mux1/1
  PS-Simulink Converter3/1 -> Mux2/3
  PS-Simulink Converter6/1 -> Mux2/2
  PS-Simulink Converter2/1 -> Mux2/1
  PS-Simulink Converter10/1 -> Mux3/2
  PS-Simulink Converter8/1 -> Mux3/3
  PS-Simulink Converter7/1 -> Mux3/1
  Mux2/1 -> Bus Creator1/2
  Mux1/1 -> formPoseMat/2(posVec), Bus Creator1/1
  Mux3/1 -> Bus Creator1/3
  PS-Simulink Converter9/1 -> Mux5/1
  PS-Simulink Converter14/1 -> Mux5/2
  PS-Simulink Converter13/1 -> Mux5/3
  Mux5/1 -> Bus Creator/3
  PS-Simulink Converter15/1 -> Mux6/2
  PS-Simulink Converter12/1 -> Mux6/3
  Mux6/1 -> Bus Creator/4
  PS-Simulink Converter11/1 -> Mux6/1
  PS-Simulink Converter16/1 -> Bus Creator/1, MATLAB Function/1(qin)
  QuatToEuler321/1(euler) -> Bus Creator/2
  Bus Creator/1 -> Bus Creator2/1
  Bus Creator1/1 -> Bus Creator2/2
  Bus Creator2/1 -> State_Bus/1
  MATLAB Function/1(qout) -> QuatToDCM/1(q), QuatToEuler321/1(q)
  QuatToDCM/1(mat) -> formPoseMat/1(rotMat)
  formPoseMat/1(mat) -> Bus Creator2/3
  connections:
  Transform Sensor/LConn1 -- B/RConn1
  Transform Sensor/RConn1 -- F/RConn1
  Transform Sensor/RConn9 -- PS-Simulink Converter1/LConn1
  Transform Sensor/RConn10 -- PS-Simulink Converter5/LConn1
  Transform Sensor/RConn11 -- PS-Simulink Converter4/LConn1
  PS-Simulink Converter3/LConn1 -- Transform Sensor/RConn14
  PS-Simulink Converter6/LConn1 -- Transform Sensor/RConn13
  PS-Simulink Converter2/LConn1 -- Transform Sensor/RConn12
  Transform Sensor/RConn17 -- PS-Simulink Converter8/LConn1
  Transform Sensor/RConn15 -- PS-Simulink Converter7/LConn1
  Transform Sensor/RConn16 -- PS-Simulink Converter10/LConn1
  Transform Sensor/RConn8 -- PS-Simulink Converter12/LConn1
  Transform Sensor/RConn5 -- PS-Simulink Converter13/LConn1
  Transform Sensor/RConn4 -- PS-Simulink Converter14/LConn1
  Transform Sensor/RConn3 -- PS-Simulink Converter9/LConn1
  Transform Sensor/RConn7 -- PS-Simulink Converter15/LConn1
  Transform Sensor/RConn6 -- PS-Simulink Converter11/LConn1
  Transform Sensor/RConn2 -- PS-Simulink Converter16/LConn1

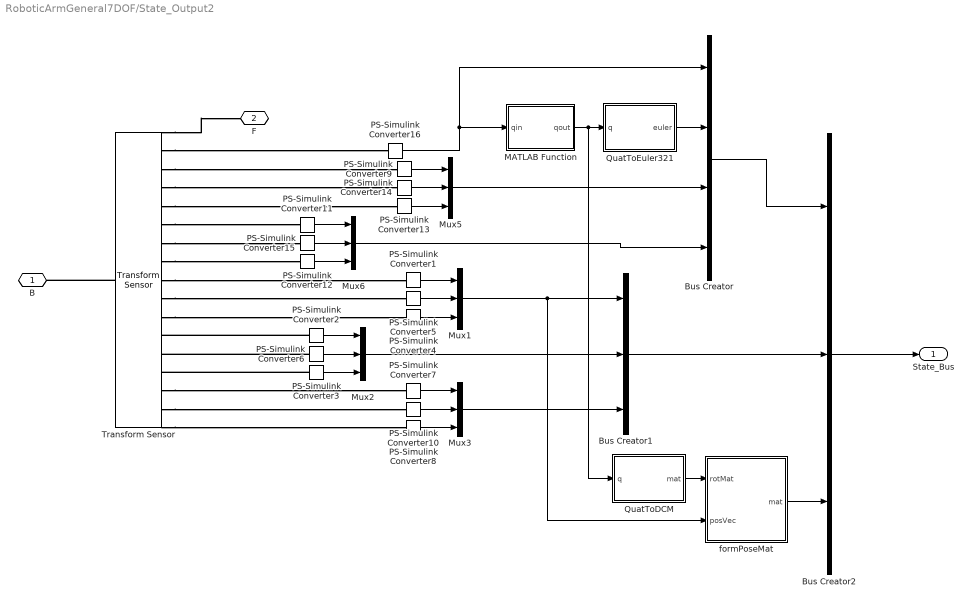
== system RoboticArmGeneral7DOF/State_Output2 ==
  Bus Creator : BusCreator  Inputs=4  OutDataTypeStr=Bus: RotStateBus
      settings: InheritFromInputs=off
  Bus Creator1 : BusCreator  Inputs=3  OutDataTypeStr=Bus: TransStateBus
      settings: InheritFromInputs=off
  Bus Creator2 : BusCreator  Inputs=3  OutDataTypeStr=Bus: StateBus
      settings: InheritFromInputs=off
  MATLAB Function : MATLAB Function  TreatAsAtomicUnit=on
  Mux{1..3,5..6} (5 alike) : Mux  Inputs=3
  PS-Simulink Converter{1..16} (16 alike) : nesl_utility/PS-Simulink Converter  PhysicalDomain=network_engine_domain  SubClassName=ps_output  LeftPortType=input  RightPortType=output  PseudoPeriodic=off  Frequencies=[]  VectorFormat=1-D array  Unit=inherit  AffineConversion=off
      settings: SourceProductBaseCode=SS,PW,VE
  QuatToDCM : MATLAB Function  TreatAsAtomicUnit=on
  QuatToEuler321 : MATLAB Function  TreatAsAtomicUnit=on
  Transform Sensor : sm_lib/Frames and Transforms/Transform Sensor  MeasurementFrame=World  SenseAngle=off  SenseAxis=off  SenseAngle1=off  SenseAngle2=off  SenseAngle3=off  SenseQ=on  SenseR=off  SenseOmegaX=on  SenseOmegaY=on  SenseOmegaZ=on  SenseOmega1=off  SenseOmega2=off  SenseOmega3=off  SenseQDot=off  SenseRDot=off  SenseAlphaX=on  SenseAlphaY=on  SenseAlphaZ=on  SenseAlpha1=off  SenseAlpha2=off  SenseAlpha3=off  SenseQDDot=off  SenseRDDot=off  SenseX=on  SenseY=on  SenseZ=on  SenseRad=off  SenseAzim=off  SenseDist=off  SenseInc=off  SenseXDot=on  SenseYDot=on  SenseZDot=on  SenseRadDot=off  SenseAzimDot=off  SenseDistDot=off  SenseIncDot=off  SenseXDDot=on  SenseYDDot=on  SenseZDDot=on  SenseRadDDot=off  SenseAzimDDot=off  SenseDistDDot=off  SenseIncDDot=off
  formPoseMat : MATLAB Function  TreatAsAtomicUnit=on
  B : PMIOPort  Side=Left
  F : PMIOPort  Port=2  Side=Right
  State_Bus : Outport
  wires:
  formPoseMat/1(mat) -> Bus Creator2/3
  QuatToDCM/1(mat) -> formPoseMat/1(rotMat)
  MATLAB Function/1(qout) -> QuatToEuler321/1(q), QuatToDCM/1(q)
  Bus Creator2/1 -> State_Bus/1
  Bus Creator1/1 -> Bus Creator2/2
  Bus Creator/1 -> Bus Creator2/1
  QuatToEuler321/1(euler) -> Bus Creator/2
  PS-Simulink Converter16/1 -> MATLAB Function/1(qin), Bus Creator/1
  PS-Simulink Converter11/1 -> Mux6/1
  Mux6/1 -> Bus Creator/4
  PS-Simulink Converter12/1 -> Mux6/3
  PS-Simulink Converter15/1 -> Mux6/2
  Mux5/1 -> Bus Creator/3
  PS-Simulink Converter13/1 -> Mux5/3
  PS-Simulink Converter14/1 -> Mux5/2
  PS-Simulink Converter9/1 -> Mux5/1
  Mux3/1 -> Bus Creator1/3
  Mux1/1 -> Bus Creator1/1, formPoseMat/2(posVec)
  Mux2/1 -> Bus Creator1/2
  PS-Simulink Converter7/1 -> Mux3/1
  PS-Simulink Converter8/1 -> Mux3/3
  PS-Simulink Converter10/1 -> Mux3/2
  PS-Simulink Converter2/1 -> Mux2/1
  PS-Simulink Converter6/1 -> Mux2/2
  PS-Simulink Converter3/1 -> Mux2/3
  PS-Simulink Converter1/1 -> Mux1/1
  PS-Simulink Converter5/1 -> Mux1/2
  PS-Simulink Converter4/1 -> Mux1/3
  connections:
  Transform Sensor/RConn2 -- PS-Simulink Converter16/LConn1
  Transform Sensor/RConn6 -- PS-Simulink Converter11/LConn1
  Transform Sensor/RConn7 -- PS-Simulink Converter15/LConn1
  Transform Sensor/RConn3 -- PS-Simulink Converter9/LConn1
  Transform Sensor/RConn4 -- PS-Simulink Converter14/LConn1
  Transform Sensor/RConn5 -- PS-Simulink Converter13/LConn1
  Transform Sensor/RConn8 -- PS-Simulink Converter12/LConn1
  Transform Sensor/RConn16 -- PS-Simulink Converter10/LConn1
  Transform Sensor/RConn15 -- PS-Simulink Converter7/LConn1
  Transform Sensor/RConn17 -- PS-Simulink Converter8/LConn1
  PS-Simulink Converter2/LConn1 -- Transform Sensor/RConn12
  PS-Simulink Converter6/LConn1 -- Transform Sensor/RConn13
  PS-Simulink Converter3/LConn1 -- Transform Sensor/RConn14
  Transform Sensor/RConn11 -- PS-Simulink Converter4/LConn1
  Transform Sensor/RConn10 -- PS-Simulink Converter5/LConn1
  Transform Sensor/RConn9 -- PS-Simulink Converter1/LConn1
  Transform Sensor/RConn1 -- F/RConn1
  Transform Sensor/LConn1 -- B/RConn1

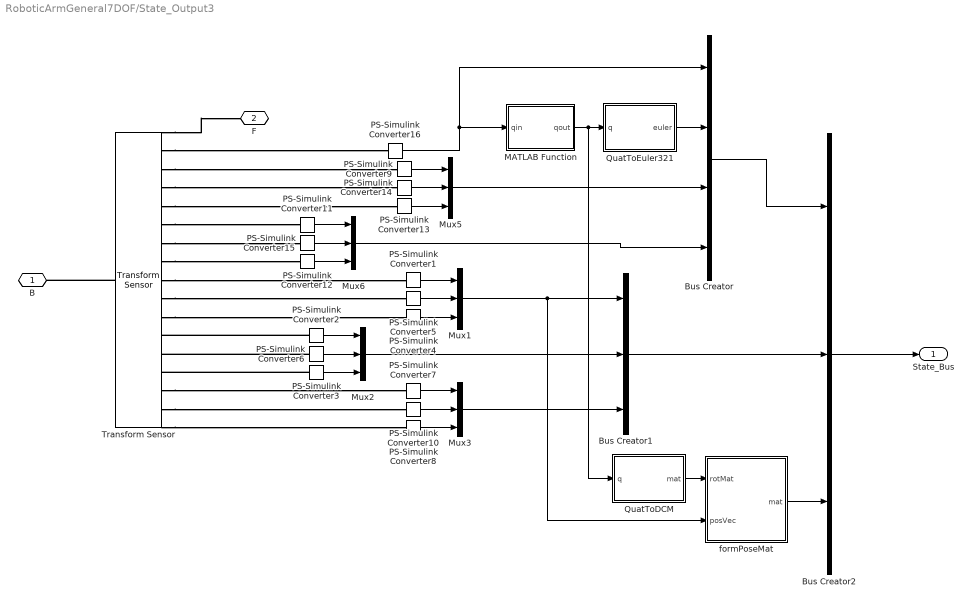
== system RoboticArmGeneral7DOF/State_Output3 ==
  Bus Creator : BusCreator  Inputs=4  OutDataTypeStr=Bus: RotStateBus
      settings: InheritFromInputs=off
  Bus Creator1 : BusCreator  Inputs=3  OutDataTypeStr=Bus: TransStateBus
      settings: InheritFromInputs=off
  Bus Creator2 : BusCreator  Inputs=3  OutDataTypeStr=Bus: StateBus
      settings: InheritFromInputs=off
  MATLAB Function : MATLAB Function  TreatAsAtomicUnit=on
  Mux{1..3,5..6} (5 alike) : Mux  Inputs=3
  PS-Simulink Converter{1..16} (16 alike) : nesl_utility/PS-Simulink Converter  PhysicalDomain=network_engine_domain  SubClassName=ps_output  LeftPortType=input  RightPortType=output  PseudoPeriodic=off  Frequencies=[]  VectorFormat=1-D array  Unit=inherit  AffineConversion=off
      settings: SourceProductBaseCode=SS,PW,VE
  QuatToDCM : MATLAB Function  TreatAsAtomicUnit=on
  QuatToEuler321 : MATLAB Function  TreatAsAtomicUnit=on
  Transform Sensor : sm_lib/Frames and Transforms/Transform Sensor  MeasurementFrame=World  SenseAngle=off  SenseAxis=off  SenseAngle1=off  SenseAngle2=off  SenseAngle3=off  SenseQ=on  SenseR=off  SenseOmegaX=on  SenseOmegaY=on  SenseOmegaZ=on  SenseOmega1=off  SenseOmega2=off  SenseOmega3=off  SenseQDot=off  SenseRDot=off  SenseAlphaX=on  SenseAlphaY=on  SenseAlphaZ=on  SenseAlpha1=off  SenseAlpha2=off  SenseAlpha3=off  SenseQDDot=off  SenseRDDot=off  SenseX=on  SenseY=on  SenseZ=on  SenseRad=off  SenseAzim=off  SenseDist=off  SenseInc=off  SenseXDot=on  SenseYDot=on  SenseZDot=on  SenseRadDot=off  SenseAzimDot=off  SenseDistDot=off  SenseIncDot=off  SenseXDDot=on  SenseYDDot=on  SenseZDDot=on  SenseRadDDot=off  SenseAzimDDot=off  SenseDistDDot=off  SenseIncDDot=off
  formPoseMat : MATLAB Function  TreatAsAtomicUnit=on
  B : PMIOPort  Side=Left
  F : PMIOPort  Port=2  Side=Right
  State_Bus : Outport
  wires:
  PS-Simulink Converter4/1 -> Mux1/3
  PS-Simulink Converter5/1 -> Mux1/2
  PS-Simulink Converter1/1 -> Mux1/1
  PS-Simulink Converter3/1 -> Mux2/3
  PS-Simulink Converter6/1 -> Mux2/2
  PS-Simulink Converter2/1 -> Mux2/1
  PS-Simulink Converter10/1 -> Mux3/2
  PS-Simulink Converter8/1 -> Mux3/3
  PS-Simulink Converter7/1 -> Mux3/1
  Mux2/1 -> Bus Creator1/2
  Mux1/1 -> formPoseMat/2(posVec), Bus Creator1/1
  Mux3/1 -> Bus Creator1/3
  PS-Simulink Converter9/1 -> Mux5/1
  PS-Simulink Converter14/1 -> Mux5/2
  PS-Simulink Converter13/1 -> Mux5/3
  Mux5/1 -> Bus Creator/3
  PS-Simulink Converter15/1 -> Mux6/2
  PS-Simulink Converter12/1 -> Mux6/3
  Mux6/1 -> Bus Creator/4
  PS-Simulink Converter11/1 -> Mux6/1
  PS-Simulink Converter16/1 -> Bus Creator/1, MATLAB Function/1(qin)
  QuatToEuler321/1(euler) -> Bus Creator/2
  Bus Creator/1 -> Bus Creator2/1
  Bus Creator1/1 -> Bus Creator2/2
  Bus Creator2/1 -> State_Bus/1
  MATLAB Function/1(qout) -> QuatToDCM/1(q), QuatToEuler321/1(q)
  QuatToDCM/1(mat) -> formPoseMat/1(rotMat)
  formPoseMat/1(mat) -> Bus Creator2/3
  connections:
  Transform Sensor/LConn1 -- B/RConn1
  Transform Sensor/RConn1 -- F/RConn1
  Transform Sensor/RConn9 -- PS-Simulink Converter1/LConn1
  Transform Sensor/RConn10 -- PS-Simulink Converter5/LConn1
  Transform Sensor/RConn11 -- PS-Simulink Converter4/LConn1
  PS-Simulink Converter3/LConn1 -- Transform Sensor/RConn14
  PS-Simulink Converter6/LConn1 -- Transform Sensor/RConn13
  PS-Simulink Converter2/LConn1 -- Transform Sensor/RConn12
  Transform Sensor/RConn17 -- PS-Simulink Converter8/LConn1
  Transform Sensor/RConn15 -- PS-Simulink Converter7/LConn1
  Transform Sensor/RConn16 -- PS-Simulink Converter10/LConn1
  Transform Sensor/RConn8 -- PS-Simulink Converter12/LConn1
  Transform Sensor/RConn5 -- PS-Simulink Converter13/LConn1
  Transform Sensor/RConn4 -- PS-Simulink Converter14/LConn1
  Transform Sensor/RConn3 -- PS-Simulink Converter9/LConn1
  Transform Sensor/RConn7 -- PS-Simulink Converter15/LConn1
  Transform Sensor/RConn6 -- PS-Simulink Converter11/LConn1
  Transform Sensor/RConn2 -- PS-Simulink Converter16/LConn1

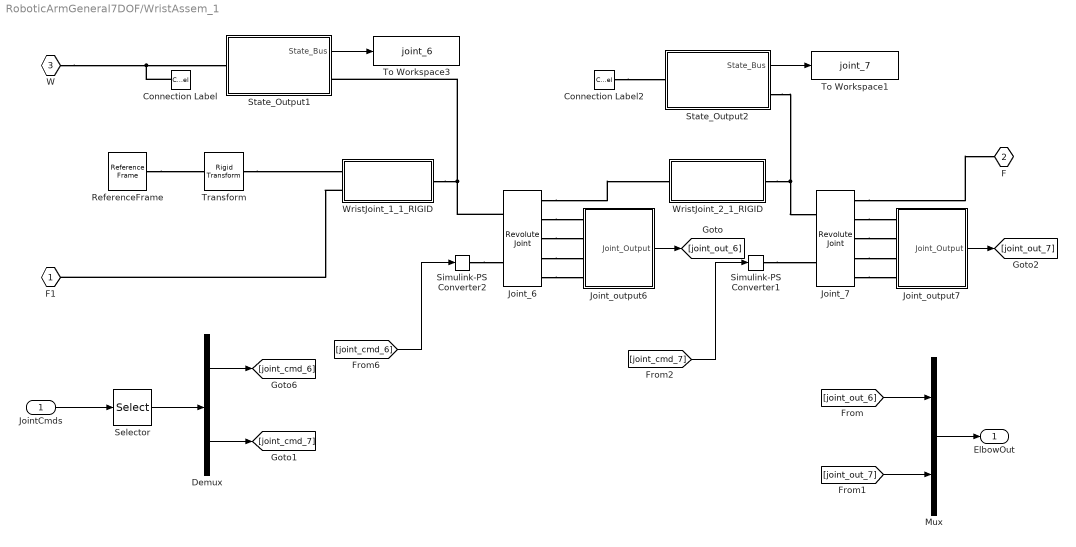
== system RoboticArmGeneral7DOF/WristAssem_1 ==
  JointCmds : Inport
  Connection Label : ConnectionLabel  Label=World
  Connection Label2 : ConnectionLabel  Label=World
  Demux : Demux  Outputs=2
  Joint_6 : sm_lib/Joints/Revolute Joint  JointMode=Normal  SenseConstraintForce=off  SenseConstraintForceX=off  SenseConstraintForceY=off  SenseConstraintForceZ=off  SenseConstraintTorque=off  SenseConstraintTorqueX=off  SenseConstraintTorqueY=off  SenseConstraintTorqueZ=off  SenseTotalForce=off  SenseTotalForceX=off  SenseTotalForceY=off  SenseTotalForceZ=off  SenseTotalTorque=on  SenseTotalTorqueX=off  SenseTotalTorqueY=off  SenseTotalTorqueZ=off  CompositeWrenchDir=FollowerOnBase  CompositeWrenchFrame=BaseFrame  EquilibriumPosition=0  EquilibriumPositionUnits=deg  SpringStiffness=0  SpringStiffnessUnits=N*m/deg  DampingCoefficient=0  DampingCoefficientUnits=N*m/(deg/s)  TorqueActuationMode=InputTorque  MotionActuationMode=ComputedMotion  SensePosition=on  SenseVelocity=on  SenseAcceleration=on  SenseTorqueForce=off  SenseLowerLimitTorqueForce=off  SenseUpperLimitTorqueForce=off  LowerLimitSpecify=off  LowerLimitBound=-90  LowerLimitBoundUnits=deg  LowerLimitStiffness=1e4  LowerLimitStiffnessUnits=N*m/deg  LowerLimitDamping=10  LowerLimitDampingUnits=N*m/(deg/s)  LowerLimitTransitionRegionWidth=0.1  LowerLimitTransitionRegionWidthUnits=deg  UpperLimitSpecify=off  UpperLimitBound=90  UpperLimitBoundUnits=deg  UpperLimitStiffness=1e4  UpperLimitStiffnessUnits=N*m/deg  UpperLimitDamping=10  UpperLimitDampingUnits=N*m/(deg/s)  UpperLimitTransitionRegionWidth=0.1  UpperLimitTransitionRegionWidthUnits=deg  PositionTargetSpecify=on  PositionTargetPriority=Low  PositionTargetValue=smiData.RevoluteJoint(6).Rz.Pos  PositionTargetValueUnits=deg  VelocityTargetSpecify=off  VelocityTargetPriority=High  VelocityTargetValue=0  VelocityTargetValueUnits=deg/s
  Joint_7 : sm_lib/Joints/Revolute Joint  JointMode=Normal  SenseConstraintForce=off  SenseConstraintForceX=off  SenseConstraintForceY=off  SenseConstraintForceZ=off  SenseConstraintTorque=off  SenseConstraintTorqueX=off  SenseConstraintTorqueY=off  SenseConstraintTorqueZ=off  SenseTotalForce=off  SenseTotalForceX=off  SenseTotalForceY=off  SenseTotalForceZ=off  SenseTotalTorque=on  SenseTotalTorqueX=off  SenseTotalTorqueY=off  SenseTotalTorqueZ=off  CompositeWrenchDir=FollowerOnBase  CompositeWrenchFrame=BaseFrame  EquilibriumPosition=0  EquilibriumPositionUnits=deg  SpringStiffness=0  SpringStiffnessUnits=N*m/deg  DampingCoefficient=0  DampingCoefficientUnits=N*m/(deg/s)  TorqueActuationMode=InputTorque  MotionActuationMode=ComputedMotion  SensePosition=on  SenseVelocity=on  SenseAcceleration=on  SenseTorqueForce=off  SenseLowerLimitTorqueForce=off  SenseUpperLimitTorqueForce=off  LowerLimitSpecify=off  LowerLimitBound=-90  LowerLimitBoundUnits=deg  LowerLimitStiffness=1e4  LowerLimitStiffnessUnits=N*m/deg  LowerLimitDamping=10  LowerLimitDampingUnits=N*m/(deg/s)  LowerLimitTransitionRegionWidth=0.1  LowerLimitTransitionRegionWidthUnits=deg  UpperLimitSpecify=off  UpperLimitBound=90  UpperLimitBoundUnits=deg  UpperLimitStiffness=1e4  UpperLimitStiffnessUnits=N*m/deg  UpperLimitDamping=10  UpperLimitDampingUnits=N*m/(deg/s)  UpperLimitTransitionRegionWidth=0.1  UpperLimitTransitionRegionWidthUnits=deg  PositionTargetSpecify=on  PositionTargetPriority=Low  PositionTargetValue=smiData.RevoluteJoint(7).Rz.Pos  PositionTargetValueUnits=deg  VelocityTargetSpecify=off  VelocityTargetPriority=High  VelocityTargetValue=0  VelocityTargetValueUnits=deg/s
  Joint_output6 : Subsystem
  Joint_output7 : Subsystem
  Mux : Mux  Inputs=2
  ReferenceFrame : sm_lib/Frames and Transforms/Reference Frame
  Selector : Selector  InputPortWidth=7  IndexOptions=Index vector (dialog)  Indices=[6 7]  OutputSizes=1
  Simulink-PS Converter1 : nesl_utility/Simulink-PS Converter  PhysicalDomain=network_engine_domain  SubClassName=ps_input  LeftPortType=input  RightPortType=output  PseudoPeriodic=off  Frequencies=[]  NoiseDistribution=none  NoiseParameters=[]  Unit=1  AffineConversion=off  FilteringAndDerivatives=filter  SimscapeFilterOrder=2  InputFilterTimeConstant=0.001  UdotUserProvided=0
      settings: SourceProductBaseCode=SS,PW,VE
  Simulink-PS Converter2 : nesl_utility/Simulink-PS Converter  PhysicalDomain=network_engine_domain  SubClassName=ps_input  LeftPortType=input  RightPortType=output  PseudoPeriodic=off  Frequencies=[]  NoiseDistribution=none  NoiseParameters=[]  Unit=1  AffineConversion=off  FilteringAndDerivatives=filter  SimscapeFilterOrder=2  InputFilterTimeConstant=0.001  UdotUserProvided=0
      settings: SourceProductBaseCode=SS,PW,VE
  State_Output1 : Subsystem
  State_Output2 : Subsystem
  To Workspace1 : ToWorkspace  VariableName=joint_7  SaveFormat=Timeseries  SampleTime=-1
  To Workspace3 : ToWorkspace  VariableName=joint_6  SaveFormat=Timeseries  SampleTime=-1
  Transform : sm_lib/Frames and Transforms/Rigid Transform  TranslationMethod=Cartesian  TranslationStandardOffset=0  TranslationLengthUnit=m  TranslationStandardAxis=+Z  TranslationCartesianOffset=smiData.RigidTransform(24).translation  TranslationROffset=0  TranslationROffsetUnits=m  TranslationZOffset=0  TranslationZOffsetUnits=m  TranslationThetaOffset=0  TranslationThetaOffsetUnits=deg  RotationMethod=ArbitraryAxis  RotationAngleUnits=rad  RotationStandardAxis=+Z  RotationAngle=smiData.RigidTransform(24).angle  RotationArbitraryAxis=smiData.RigidTransform(24).axis  FollAlignAxisA=+X  BaseAlignAxisA=+Y  FollAlignAxisB=+Y  BaseAlignAxisB=+Z  RotationSequenceAxes=FollowerAxes  RotationSequence=XYX  RotationSequenceAngles=[0 0 0]  RotationSequenceAnglesUnits=deg  RotationMatrix=[1 0 0; 0 1 0; 0 0 1]
  WristJoint_1_1_RIGID : Subsystem
  WristJoint_2_1_RIGID : Subsystem
  F1 : PMIOPort  Side=Left
  F : PMIOPort  Port=2  Side=Right
  W : PMIOPort  Port=3  Side=Left
  ElbowOut : Outport
  wires:
  State_Output2/1(State_Bus) -> To Workspace1/1
  Joint_output6/1(Joint_Output) -> [joint_out_6]
  [joint_cmd_6] -> Simulink-PS Converter2/1
  Joint_output7/1(Joint_Output) -> [joint_out_7]
  [joint_cmd_7] -> Simulink-PS Converter1/1
  State_Output1/1(State_Bus) -> To Workspace3/1
  [joint_out_7] -> Mux/2
  [joint_out_6] -> Mux/1
  Mux/1 -> ElbowOut/1
  JointCmds/1 -> Selector/1
  Demux/2 -> [joint_cmd_7]
  Demux/1 -> [joint_cmd_6]
  Selector/1 -> Demux/1
  connections:
  Connection Label2/LConn1 -- State_Output2/LConn1
  Joint_7/RConn1 -- F/RConn1
  State_Output2/RConn1 -- Joint_7/LConn1 -- WristJoint_2_1_RIGID/RConn1
  Joint_6/RConn1 -- WristJoint_2_1_RIGID/LConn1
  Joint_6/RConn5 -- Joint_output6/LConn4
  Joint_7/RConn3 -- Joint_output7/LConn2
  Simulink-PS Converter1/RConn1 -- Joint_7/LConn2
  Joint_6/RConn4 -- Joint_output6/LConn3
  Joint_6/RConn2 -- Joint_output6/LConn1
  Joint_7/RConn4 -- Joint_output7/LConn3
  Joint_6/RConn3 -- Joint_output6/LConn2
  Simulink-PS Converter2/RConn1 -- Joint_6/LConn2
  Joint_7/RConn5 -- Joint_output7/LConn4
  Joint_7/RConn2 -- Joint_output7/LConn1
  Connection Label/LConn1 -- W/RConn1 -- State_Output1/LConn1
  ReferenceFrame/RConn1 -- Transform/LConn1
  Transform/RConn1 -- WristJoint_1_1_RIGID/LConn1
  WristJoint_1_1_RIGID/LConn2 -- F1/RConn1
  Joint_6/LConn1 -- WristJoint_1_1_RIGID/RConn1 -- State_Output1/RConn1

== system RoboticArmGeneral7DOF/ElbowAssem_1/ElbowJoint_1_1_RIGID ==
  ReferenceFrame : sm_lib/Frames and Transforms/Reference Frame
  Solid : sm_lib/Body Elements/File Solid  ExtGeomFileName=ElbowJoint_1_Default_sldprt.STEP  UnitType=FromFile  ExtGeomFileUnits=m  StepReaderType=HEX  ExportConvexHullGeometry=off  InertiaType=Custom  Mass=smiData.Solid(4).mass  MassUnits=kg  CenterOfMass=smiData.Solid(4).CoM  CenterOfMassUnits=m  MomentsOfInertia=smiData.Solid(4).MoI  MomentsOfInertiaUnits=kg*m^2  ProductsOfInertia=smiData.Solid(4).PoI  ProductsOfInertiaUnits=kg*m^2  BasedOnType=DensityFromFile  Density=1000  DensityUnits=kg/m^3  DoExposeReferenceFrame=on  SerializedFrames=<Frames/>  GraphicType=FromGeometry  MarkerShape=Sphere  MarkerSize=10  GraphicVisPropType=SimpleVisualProperties  GraphicDiffuseColor=smiData.Solid(4).color  GraphicSpecularColor=[0.5 0.5 0.5 1.0]  GraphicAmbientColor=[0.15 0.15 0.15 1.0]  GraphicEmissiveColor=[0.0 0.0 0.0 1.0]  GraphicShininess=75  GraphicOpacity=smiData.Solid(4).opacity
  Transform : sm_lib/Frames and Transforms/Rigid Transform  TranslationMethod=Cartesian  TranslationStandardOffset=0  TranslationLengthUnit=m  TranslationStandardAxis=+Z  TranslationCartesianOffset=smiData.RigidTransform(1).translation  TranslationROffset=0  TranslationROffsetUnits=m  TranslationZOffset=0  TranslationZOffsetUnits=m  TranslationThetaOffset=0  TranslationThetaOffsetUnits=deg  RotationMethod=ArbitraryAxis  RotationAngleUnits=rad  RotationStandardAxis=+Z  RotationAngle=smiData.RigidTransform(1).angle  RotationArbitraryAxis=smiData.RigidTransform(1).axis  FollAlignAxisA=+X  BaseAlignAxisA=+Y  FollAlignAxisB=+Y  BaseAlignAxisB=+Z  RotationSequenceAxes=FollowerAxes  RotationSequence=XYX  RotationSequenceAngles=[0 0 0]  RotationSequenceAnglesUnits=deg  RotationMatrix=[1 0 0; 0 1 0; 0 0 1]
  Transform1 : sm_lib/Frames and Transforms/Rigid Transform  TranslationMethod=Cartesian  TranslationStandardOffset=0  TranslationLengthUnit=m  TranslationStandardAxis=+Z  TranslationCartesianOffset=smiData.RigidTransform(3).translation  TranslationROffset=0  TranslationROffsetUnits=m  TranslationZOffset=0  TranslationZOffsetUnits=m  TranslationThetaOffset=0  TranslationThetaOffsetUnits=deg  RotationMethod=ArbitraryAxis  RotationAngleUnits=rad  RotationStandardAxis=+Z  RotationAngle=smiData.RigidTransform(3).angle  RotationArbitraryAxis=smiData.RigidTransform(3).axis  FollAlignAxisA=+X  BaseAlignAxisA=+Y  FollAlignAxisB=+Y  BaseAlignAxisB=+Z  RotationSequenceAxes=FollowerAxes  RotationSequence=XYX  RotationSequenceAngles=[0 0 0]  RotationSequenceAnglesUnits=deg  RotationMatrix=[1 0 0; 0 1 0; 0 0 1]
  F : PMIOPort  Side=Left
  J4_1 : PMIOPort  Port=2  Side=Right
  connections:
  Transform1/RConn1 -- F/RConn1
  Transform/RConn1 -- J4_1/RConn1
  Transform1/LConn1 -- Transform/LConn1 -- ReferenceFrame/RConn1 -- Solid/RConn1
